simulink model "ThreeINVTRECT2025"  (R2024a)
settings: Solver=FixedStepAuto  StartTime=0.0  StopTime=0.3  FixedStep=2e-7  RelTol=1e-3
libraries: spsSeriesRLCBranchLib x27, spsCurrentMeasurementLib x5, spsUniversalBridgeLib x4, spsMeanLib x3, simulink x3, spsVoltageMeasurementLib x3, spsDCVoltageSourceLib x2, spsMutualInductanceLib x2, spsRMSLib x2, spsTHDLib x2, spspowerguiLib x1
settings Model: SimulationMode=accelerator  Creator=abc6820292  LastModifiedBy=50803
settings SolverCC: ZeroCrossControl=EnableAll  ZeroCrossAlgorithm=Adaptive
settings DebuggingCC: UnconnectedInputMsg=warning  UnconnectedOutputMsg=warning  UnconnectedLineMsg=warning
settings ModelReferenceCC: EnableRefExpFcnMdlSchedulingChecks=on
settings SFSimCC: SimTargetLang=C++
settings RTWCC: BuildConfiguration=Faster Runs  GPUComputeCapability=3.5  DLArmComputeVersion=19.05

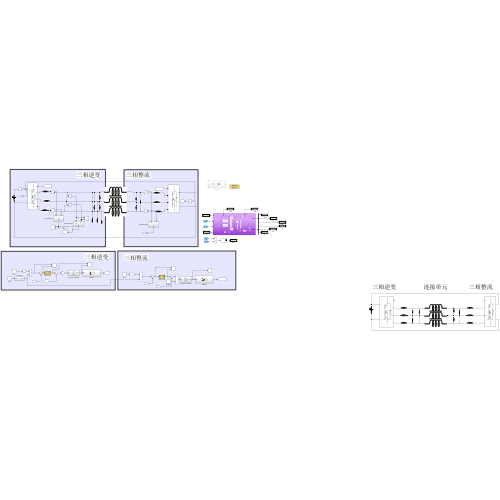
[thumbnail: Simulink's stored preview of the top-level diagram]
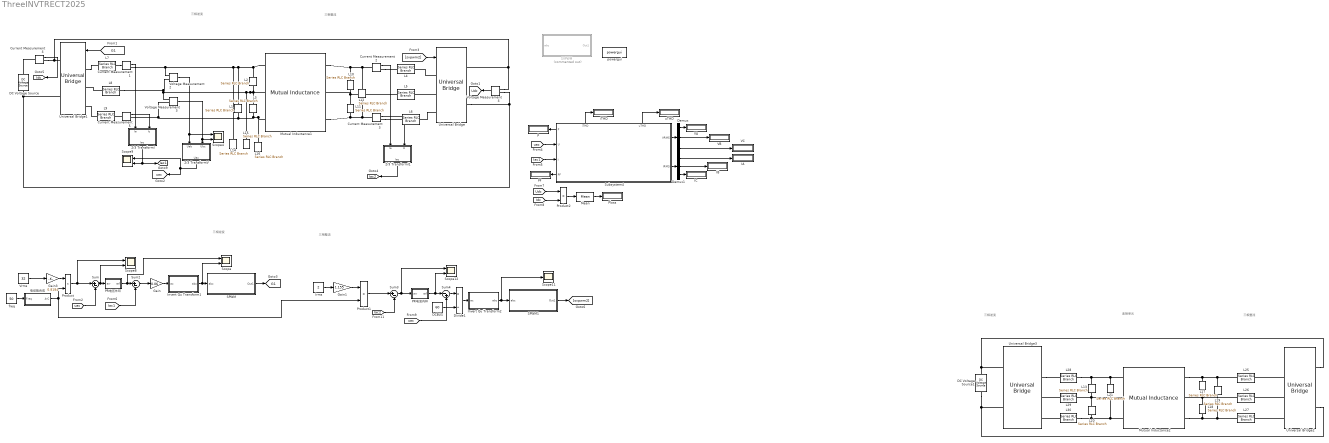
== system ThreeINVTRECT2025 ==
  note: 连接单元
  note: 三相逆变
  note: 三相逆变
  note: 三相整流
  note: 三相整流
  note: 三相逆变
  note: 三相整流
  2/3 TransformI : Subsystem
  2/3 TransformI1 : Subsystem
  2/3 TransformV : Subsystem
  Current Measurement{1..5} (5 alike) : spsCurrentMeasurementLib/Current Measurement  PhasorSimulation=off  OutputType=Complex  PSBequivalent=0
  DC Voltage Source : spsDCVoltageSourceLib/DC Voltage Source  Amplitude=60  Measurements=None
  DC Voltage Source1 : spsDCVoltageSourceLib/DC Voltage Source  Amplitude=60  Measurements=None
  DCBUS : Constant  Value=60
  Demux : Demux  Outputs=3
  Demux1 : Demux  Outputs=3
  Divide1 : Product  Inputs=*/
  Gain : Gain  Gain=0.06
  Gain1 : Gain  Gain=1.155
  Gain3 : Gain  Gain=0.8184
  IA : Display
      settings: Format=bank
  IB : Display
      settings: Format=bank
  IC : Display
      settings: Format=bank
  Invert Qu Transform1 : Subsystem
  Invert Qu Transform2 : Subsystem
  Irms : Constant  Value=2
  L{1..3,10..13,17..21} (12 alike) : spsSeriesRLCBranchLib/Series RLC Branch  LConnTagsString=__new0  RConnTagsString=__new0  BranchType=C  Resistance=16  Inductance=2e-3  SetiL0=off  InitialCurrent=0  Capacitance=2.2e-6  Setx0=off  InitialVoltage=0  Measurements=None
  L14 : spsSeriesRLCBranchLib/Series RLC Branch  LConnTagsString=__new0  RConnTagsString=__new0  BranchType=R  Resistance=16  Inductance=2e-3  SetiL0=off  InitialCurrent=0  Capacitance=2.2e-6  Setx0=off  InitialVoltage=0  Measurements=None
  L15 : spsSeriesRLCBranchLib/Series RLC Branch  LConnTagsString=__new0  RConnTagsString=__new0  BranchType=R  Resistance=16  Inductance=2e-3  SetiL0=off  InitialCurrent=0  Capacitance=2.2e-6  Setx0=off  InitialVoltage=0  Measurements=None
  L16 : spsSeriesRLCBranchLib/Series RLC Branch  LConnTagsString=__new0  RConnTagsString=__new0  BranchType=R  Resistance=16  Inductance=2e-3  SetiL0=off  InitialCurrent=0  Capacitance=2.2e-6  Setx0=off  InitialVoltage=0  Measurements=None
  L{4..9,25..30} (12 alike) : spsSeriesRLCBranchLib/Series RLC Branch  LConnTagsString=__new0  RConnTagsString=__new0  BranchType=L  Resistance=1  Inductance=7e-4  SetiL0=off  InitialCurrent=0  Capacitance=2e-3  Setx0=off  InitialVoltage=0  Measurements=None
  Mean : spsMeanLib/Mean  Freq=50  Vinit=0  Ts=0
  Mutual Inductance1 : spsMutualInductanceLib/Mutual Inductance  LConnTagsString=a|b|c  RConnTagsString=A|B|C  TypeOfMutual=Two or three windings with equal mutual terms  NumberOfWindings=3  SelfImpedance1=[0.01 1e-03]  SelfImpedance2=[0.01 1e-03]  ThreeWindings=on  SelfImpedance3=[0.01 1e-03]  MutualImpedance=[0.02 0.9e-03]  InductanceMatrix="[1.0 0.9  0.9 ;  0.9 1.0  0.9;  0.9 0.9 1.0 ] * 1e-3"  ResistanceMatrix="[1.0 0.9  0.9 ;  0.9 1.0  0.9;  0.9 0.9 1.0 ]"  Measurements=None
  Mutual Inductance2 : spsMutualInductanceLib/Mutual Inductance  LConnTagsString=a|b|c  RConnTagsString=A|B|C  TypeOfMutual=Two or three windings with equal mutual terms  NumberOfWindings=3  SelfImpedance1=[0.01 1e-03]  SelfImpedance2=[0.01 1e-03]  ThreeWindings=on  SelfImpedance3=[0.01 1e-03]  MutualImpedance=[0.02 0.9e-03]  InductanceMatrix="[1.0 0.9  0.9 ;  0.9 1.0  0.9;  0.9 0.9 1.0 ] * 1e-3"  ResistanceMatrix="[1.0 0.9  0.9 ;  0.9 1.0  0.9;  0.9 0.9 1.0 ]"  Measurements=None
  P : Display
      settings: Format=bank
  PF : Display
  PR电压外环 : Subsystem  TreatAsAtomicUnit=on  mask{Kp=1, Kr=50, Wc=5, Upper=80, Lower=-80}
  PR电流内环 : Subsystem  TreatAsAtomicUnit=on  mask{Kp=2, Kr=50, Wc=5, Upper=80, Lower=-80}
  Ploss : Display
  Product : Product
  Product1 : Product
  Product2 : Product
  SPWM : Subsystem
  SPWM1 : Subsystem
  SVPWM : Subsystem  Commented=on
  Scope{,4,8..9,12} (5 alike) : Scope  NumInputPorts=2
  Scope11 : Scope
  Subsystem4 : Subsystem
      settings: PortSchema="{\"entries\":[{\"content\":{\"sides\":[{\"content\":{\"connectorIds\":[\"Out5\",\"In1\",\"In2\",\"Out6\"]},\"type\":\"ConnectorPlacement.EquallySpacedRectSide\",\"uuid\":\"8f3b7bf1-7c44-4492-a357-aa6e3e6d66a4\"},{\"content\":{\"connectorIds\":[\"Out1\",\"Out2\"],\"side\":\"RIGHT\"},\"type\":\"ConnectorPlacement.EquallySpacedRectSide\",\"uuid\":\"7ae784cf-6bcf-4684-9c07-1770fc60c8a0\"},{\"content\":{\"connectorIds\":[\"Out3\",\"Out4\"],\"side\":\"TOP\"},\"type\":\"ConnectorPlacement.EquallySpacedRectSide\",\"uuid\":\"0e016931-6232-4ad6-afe9-572a0571336f\"},{\"content\":{\"side\":\"BOTTOM\"},\"type\":\"ConnectorPlacement.EquallySpacedRectSide\",\"uuid\":\"ef67c6ee-ba81-4705-af34-81581e7e9907\"}]},\"type\":\"ConnectorPlacement.EquallySpacedConnector\",\"uuid\":\"922af512-c0ff-443f-816c-194775a78dc8\"}],\"packageUris\":[\"http://schema.mathworks.com/mf0/Connector/R2020b\"],\"version\":\"1.0\"}"
  Sum : Sum  Inputs=|+-
  Sum2 : Sum  Inputs=|+-
  Sum3 : Sum  Inputs=|+-
  Sum4 : Sum  Inputs=|-+
  Universal Bridge{,1..3} (4 alike) : spsUniversalBridgeLib/Universal Bridge  Arms=3  SnubberResistance=1e5  SnubberCapacitance=inf  Device=MOSFET / Diodes  Ron=1e-3  Lon=0  ForwardVoltages="[  0  0  ]"  ForwardVoltage=0  GTOparameters=[ 10e-6 , 20e-6 ]  IGBTparameters=[ 1e-6 , 2e-6 ]  Measurements=None  Measurements_2=None  converterType=Rectifier
  VA : Display
      settings: Format=bank
  VB : Display
      settings: Format=bank
  VC : Display
      settings: Format=bank
  Voltage Measurement2 : spsVoltageMeasurementLib/Voltage Measurement  PhasorSimulation=off  OutputType=Complex  PSBequivalent=0
  Voltage Measurement3 : spsVoltageMeasurementLib/Voltage Measurement  PhasorSimulation=off  OutputType=Complex  PSBequivalent=0
  Voltage Measurement4 : spsVoltageMeasurementLib/Voltage Measurement  PhasorSimulation=off  OutputType=Complex  PSBequivalent=0
  Vrms : Constant  Value=32
  freq : Constant  Value=50
  iTHD : Display
  powergui : spspowerguiLib/powergui  SimulationMode=Discrete  SampleTime=2e-7  frequency=60  Iterations=50  frequencyindice=0  Pbase=100e6  ErrMax=1e-4  UnitsV=kV  UnitsW=MW  buscounter=0  FunctionMessages=off  echomessages=off  EnableUseOfTLC=off  CurrentSourceSwitches=off  DisableSnubberDevices=off  DisableRonSwitches=off  DisableVfSwitches=off  DisplayEquations=off  AutomaticDiscreteSolvers=off  SolverType=Tustin/Backward Euler (TBE)  Interpol=off  ExternalGateDelay=off  methode=off  Ts=0  x0status=blocks  SPID=off  SwTol=0  HookPort=off  NonlinearTolerance=1e-4  nMaxIteration=100  ContinueOnMaxIteration=off  RestoreLinks=warning  ResistiveCurrentMeasurement=off  Frange=[0:2:500]  Ylog=off  Xlog=on  ShowGrid=off  save=off  variable=ZData  structure=QQQQQ  ZoomFFT=off  StartTime=0.5  cycles=15  DisplayStyle=1  fundamental=50  FreqAxis=off  MaxFrequency=1000  frequencyindicesteady=1  RmsSteady=1  display=off
  uTHD : Display
  电动势合成 : Subsystem
      settings: PortSchema="{\"entries\":[{\"content\":{\"sides\":[{\"content\":{\"connectorIds\":[]},\"type\":\"ConnectorPlacement.EquallySpacedRectSide\",\"uuid\":\"ac756fcf-f6d7-466d-bb3d-287dec8ae983\"},{\"content\":{\"connectorIds\":[],\"side\":\"RIGHT\"},\"type\":\"ConnectorPlacement.EquallySpacedRectSide\",\"uuid\":\"3e1a0e91-a0b8-40c4-8839-5ebd84050a30\"},{\"content\":{\"connectorIds\":[\"In1\"],\"side\":\"TOP\"},\"type\":\"ConnectorPlacement.EquallySpacedRectSide\",\"uuid\":\"4c3986ff-483b-4975-8d50-1a8a46f35065\"},{\"content\":{\"connectorIds\":[\"Out1\"],\"side\":\"BOTTOM\"},\"type\":\"ConnectorPlacement.EquallySpacedRectSide\",\"uuid\":\"d0166e46-df65-4061-a961-140d500477a7\"}]},\"type\":\"ConnectorPlacement.EquallySpacedConnector\",\"uuid\":\"9d4b00aa-dfb1-427d-8698-7ec64c5ca012\"}],\"packageUris\":[\"http://schema.mathworks.com/mf0/Connector/R2020b\"],\"version\":\"1.0\"}"
  tag scope: G1=global, Iac1=global, Iac2=global, Idc=global, Udc=global, uac=global
  wires:
  [Iac1] -> Subsystem4/2(I)
  PR电流内环/1(ref) -> Sum4/1, Scope12/2
  [Iac2] -> Sum3/2
  Demux/3 -> VC/1
  [Iac1] -> Sum2/2
  Current Measurement5/1 -> 2/3 TransformI/2(Ic)
  Subsystem4/2(IRMS) -> Demux1/1
  2/3 TransformI/1(Iac) -> Scope9/2, [Iac1]
  [uac] -> Subsystem4/1(U)
  Subsystem4/1(VRMS) -> Demux/1
  Irms/1 -> Gain1/1
  Demux/2 -> VB/1
  2/3 TransformV/1(Uac) -> [uac], Scope9/1
  Demux/1 -> VA/1
  Subsystem4/5(P) -> P/1
  Demux1/3 -> IC/1
  SPWM1/1(Out1) -> [svpwm2]
  SPWM/1(Out1) -> [G1]
  Gain1/1 -> Product1/1
  Demux1/2 -> IB/1
  Current Measurement1/1 -> 2/3 TransformI/1(Ia)
  [G1] -> Universal Bridge1/1
  Voltage Measurement3/1 -> Scope4/2, 2/3 TransformV/2(Ubc)
  Subsystem4/6(PF) -> PF/1
  Sum3/1 -> PR电流内环/1(err), Scope12/1
  Invert Qu Transform2/1(abc) -> SPWM1/1(abc), Scope11/1
  Vrms/1 -> Gain3/1
  freq/1 -> 电动势合成/1(Freq)
  Demux1/1 -> IA/1
  Product1/1 -> Sum3/1
  电动势合成/1(A-C) -> Product/2, Product1/2
  [svpwm2] -> Universal Bridge/1
  Subsystem4/3(iTHD) -> iTHD/1
  Voltage Measurement2/1 -> Scope4/1, 2/3 TransformV/1(Uab)
  [uac] -> Sum/2
  Subsystem4/4(uTHD) -> uTHD/1
  Product/1 -> Scope8/1, Sum/1
  Voltage Measurement4/1 -> [Udc]
  Invert Qu Transform1/1(abc) -> Scope/2, SPWM/1(abc)
  Current Measurement2/1 -> 2/3 TransformI1/1(Ia)
  Current Measurement3/1 -> 2/3 TransformI1/2(Ic)
  2/3 TransformI1/1(Iac) -> [Iac2]
  Gain3/1 -> Product/1
  Current Measurement4/1 -> [Idc]
  [Idc] -> Product2/2
  [Udc] -> Product2/1
  Product2/1 -> Mean/1
  Mean/1 -> Ploss/1
  Divide1/1 -> Invert Qu Transform2/1(ac)
  Sum4/1 -> Divide1/1
  DCBUS/1 -> Divide1/2
  [uac] -> Sum4/2
  Sum/1 -> Scope8/2, PR电压外环/1(err)
  PR电压外环/1(ref) -> Scope/1, Sum2/1
  Gain/1 -> Invert Qu Transform1/1(ac)
  Sum2/1 -> Gain/1
  connections:
  L10/LConn1 -- Mutual Inductance1/RConn1 -- L12/LConn1 -- Current Measurement2/LConn1
  Current Measurement4/RConn1 -- Voltage Measurement4/LConn1 -- Universal Bridge/RConn1 -- Universal Bridge1/RConn1
  DC Voltage Source/LConn1 -- Universal Bridge1/RConn2 -- Universal Bridge/RConn2 -- Voltage Measurement4/LConn2
  Current Measurement5/RConn1 -- L16/LConn1 -- Mutual Inductance1/LConn3 -- L3/RConn1 -- L1/RConn1 -- Voltage Measurement3/LConn2
  Current Measurement3/RConn1 -- L6/LConn1
  L7/RConn1 -- Current Measurement1/LConn1
  Universal Bridge1/LConn1 -- L7/LConn1
  Universal Bridge/LConn3 -- L6/RConn1
  Universal Bridge/LConn2 -- L5/RConn1
  Current Measurement5/LConn1 -- L9/RConn1
  Current Measurement2/RConn1 -- L4/LConn1
  L9/LConn1 -- Universal Bridge1/LConn3
  Universal Bridge/LConn1 -- L4/RConn1
  L8/LConn1 -- Universal Bridge1/LConn2
  L5/LConn1 -- L11/LConn1 -- L10/RConn1 -- Mutual Inductance1/RConn2
  L14/LConn1 -- Current Measurement1/RConn1 -- Voltage Measurement2/LConn1 -- L1/LConn1 -- L2/LConn1 -- Mutual Inductance1/LConn1
  L3/LConn1 -- Mutual Inductance1/LConn2 -- L15/LConn1 -- L8/RConn1 -- Voltage Measurement2/LConn2 -- Voltage Measurement3/LConn1 -- L2/RConn1
  Current Measurement3/LConn1 -- Mutual Inductance1/RConn3 -- L11/RConn1 -- L12/RConn1
  DC Voltage Source/RConn1 -- Current Measurement4/LConn1
  Universal Bridge2/RConn1 -- DC Voltage Source1/RConn1 -- Universal Bridge3/RConn1
  L18/RConn1 -- L19/RConn1 -- L27/LConn1 -- Mutual Inductance2/RConn3
  Mutual Inductance2/RConn2 -- L18/LConn1 -- L26/LConn1 -- L17/RConn1
  Mutual Inductance2/RConn1 -- L25/LConn1 -- L19/LConn1 -- L17/LConn1
  Universal Bridge2/LConn1 -- L25/RConn1
  L30/RConn1 -- L20/RConn1 -- L21/RConn1 -- Mutual Inductance2/LConn3
  Universal Bridge2/LConn3 -- L27/RConn1
  L29/LConn1 -- Universal Bridge3/LConn2
  L30/LConn1 -- Universal Bridge3/LConn3
  Universal Bridge3/LConn1 -- L28/LConn1
  L28/RConn1 -- L13/LConn1 -- L21/LConn1 -- Mutual Inductance2/LConn1
  Universal Bridge2/LConn2 -- L26/RConn1
  DC Voltage Source1/LConn1 -- Universal Bridge2/RConn2 -- Universal Bridge3/RConn2
  Mutual Inductance2/LConn2 -- L13/RConn1 -- L20/LConn1 -- L29/RConn1

== system ThreeINVTRECT2025/2//3 TransformI ==
  Ia : Inport
  Ic : Inport  Port=2
  Mux : Mux  Inputs=2
  Iac : Outport
  wires:
  Ia/1 -> Mux/1
  Ic/1 -> Mux/2
  Mux/1 -> Iac/1

== system ThreeINVTRECT2025/2//3 TransformI1 ==
  Ia : Inport
  Ic : Inport  Port=2
  Mux : Mux  Inputs=2
  Iac : Outport
  wires:
  Mux/1 -> Iac/1
  Ic/1 -> Mux/2
  Ia/1 -> Mux/1

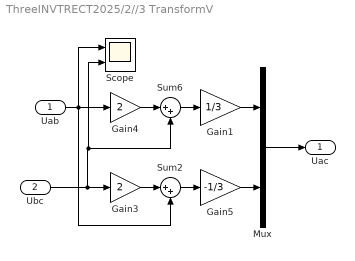
== system ThreeINVTRECT2025/2//3 TransformV ==
  Uab : Inport
  Ubc : Inport  Port=2
  Gain1 : Gain  Gain=1/3
  Gain3 : Gain  Gain=2
  Gain4 : Gain  Gain=2
  Gain5 : Gain  Gain=-1/3
  Mux : Mux  Inputs=2
  Scope : Scope  NumInputPorts=2
  Sum2 : Sum  Inputs=|++
  Sum6 : Sum  Inputs=|++
  Uac : Outport
  wires:
  Sum6/1 -> Gain1/1
  Uab/1 -> Scope/1, Sum2/2, Gain4/1
  Gain4/1 -> Sum6/1
  Ubc/1 -> Scope/2, Sum6/2, Gain3/1
  Gain3/1 -> Sum2/1
  Sum2/1 -> Gain5/1
  Gain5/1 -> Mux/2
  Gain1/1 -> Mux/1
  Mux/1 -> Uac/1

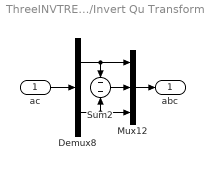
== system ThreeINVTRECT2025/Invert Qu Transform1 ==
  ac : Inport
  Demux8 : Demux  Outputs=2
  Mux12 : Mux  Inputs=3
  Sum2 : Sum  Inputs=-|-
  abc : Outport
  wires:
  Mux12/1 -> abc/1
  Demux8/2 -> Sum2/2, Mux12/3
  Sum2/1 -> Mux12/2
  ac/1 -> Demux8/1
  Demux8/1 -> Sum2/1, Mux12/1

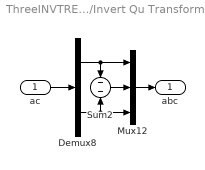
== system ThreeINVTRECT2025/Invert Qu Transform2 ==
  ac : Inport
  Demux8 : Demux  Outputs=2
  Mux12 : Mux  Inputs=3
  Sum2 : Sum  Inputs=-|-
  abc : Outport
  wires:
  Demux8/1 -> Mux12/1, Sum2/1
  ac/1 -> Demux8/1
  Sum2/1 -> Mux12/2
  Demux8/2 -> Mux12/3, Sum2/2
  Mux12/1 -> abc/1

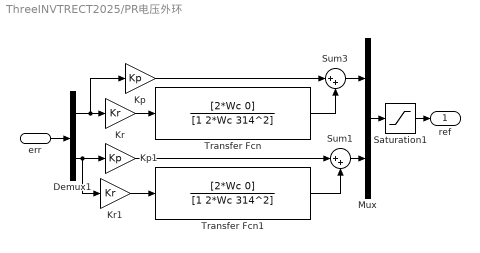
== system ThreeINVTRECT2025/PR电压外环 ==
  err : Inport
  Demux1 : Demux  Outputs=2
  Kp : Gain  Gain=Kp
  Kp1 : Gain  Gain=Kp
  Kr : Gain  Gain=Kr
  Kr1 : Gain  Gain=Kr
  Mux : Mux  Inputs=2
  Saturation1 : Saturate  UpperLimit=Upper  LowerLimit=Lower
  Sum1 : Sum  Inputs=|++
  Sum3 : Sum  Inputs=|++
  Transfer Fcn : TransferFcn  Numerator=[2*Wc 0]  Denominator=[1 2*Wc 314^2]
  Transfer Fcn1 : TransferFcn  Numerator=[2*Wc 0]  Denominator=[1 2*Wc 314^2]
  ref : Outport
  wires:
  Kp/1 -> Sum3/1
  Kr/1 -> Transfer Fcn/1
  Transfer Fcn/1 -> Sum3/2
  Demux1/1 -> Kp/1, Kr/1
  err/1 -> Demux1/1
  Demux1/2 -> Kr1/1, Kp1/1
  Kp1/1 -> Sum1/1
  Kr1/1 -> Transfer Fcn1/1
  Transfer Fcn1/1 -> Sum1/2
  Sum1/1 -> Mux/2
  Sum3/1 -> Mux/1
  Mux/1 -> Saturation1/1
  Saturation1/1 -> ref/1

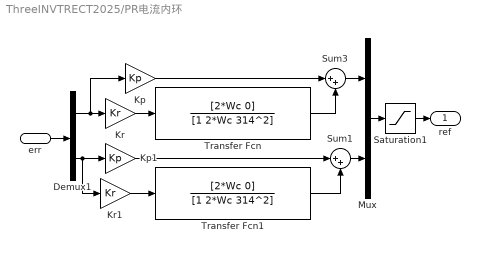
== system ThreeINVTRECT2025/PR电流内环 ==
  err : Inport
  Demux1 : Demux  Outputs=2
  Kp : Gain  Gain=Kp
  Kp1 : Gain  Gain=Kp
  Kr : Gain  Gain=Kr
  Kr1 : Gain  Gain=Kr
  Mux : Mux  Inputs=2
  Saturation1 : Saturate  UpperLimit=Upper  LowerLimit=Lower
  Sum1 : Sum  Inputs=|++
  Sum3 : Sum  Inputs=|++
  Transfer Fcn : TransferFcn  Numerator=[2*Wc 0]  Denominator=[1 2*Wc 314^2]
  Transfer Fcn1 : TransferFcn  Numerator=[2*Wc 0]  Denominator=[1 2*Wc 314^2]
  ref : Outport
  wires:
  Saturation1/1 -> ref/1
  Mux/1 -> Saturation1/1
  Sum3/1 -> Mux/1
  Sum1/1 -> Mux/2
  Transfer Fcn1/1 -> Sum1/2
  Kr1/1 -> Transfer Fcn1/1
  Kp1/1 -> Sum1/1
  Demux1/2 -> Kp1/1, Kr1/1
  err/1 -> Demux1/1
  Demux1/1 -> Kr/1, Kp/1
  Transfer Fcn/1 -> Sum3/2
  Kr/1 -> Transfer Fcn/1
  Kp/1 -> Sum3/1

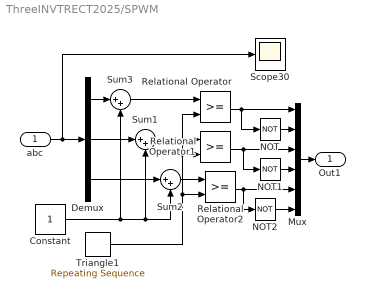
== system ThreeINVTRECT2025/SPWM ==
  abc : Inport
  Constant : Constant
  Demux : Demux  Outputs=3
  Mux : Mux  Inputs=6
  NOT : Logic  Operator=NOT  IconShape=distinctive  AllPortsSameDT=off  OutDataTypeStr=boolean
  NOT1 : Logic  Operator=NOT  IconShape=distinctive  AllPortsSameDT=off  OutDataTypeStr=boolean
  NOT2 : Logic  Operator=NOT  IconShape=distinctive  AllPortsSameDT=off  OutDataTypeStr=boolean
  Relational Operator : RelationalOperator  OutDataTypeStr=boolean  RndMeth=Simplest  InputSameDT=off
  Relational Operator1 : RelationalOperator  OutDataTypeStr=boolean  RndMeth=Simplest  InputSameDT=off
  Relational Operator2 : RelationalOperator  OutDataTypeStr=boolean  RndMeth=Simplest  InputSameDT=off
  Scope30 : Scope
  Sum1 : Sum  Inputs=|++
  Sum2 : Sum  Inputs=|++
  Sum3 : Sum  Inputs=|++
  Triangle1 : simulink/Sources/Repeating Sequence  rep_seq_t=[0 1/20000/2 1/20000]  rep_seq_y=[0 2 0]
  Out1 : Outport
  wires:
  Mux/1 -> Out1/1
  NOT2/1 -> Mux/6
  NOT1/1 -> Mux/4
  Relational Operator2/1 -> Mux/5, NOT2/1
  Relational Operator1/1 -> Mux/3, NOT1/1
  Relational Operator/1 -> Mux/1, NOT/1
  NOT/1 -> Mux/2
  Triangle1/1 -> Relational Operator/2, Relational Operator1/2, Relational Operator2/2
  abc/1 -> Scope30/1, Demux/1
  Demux/1 -> Sum3/1
  Sum3/1 -> Relational Operator/1
  Demux/2 -> Sum1/1
  Sum1/1 -> Relational Operator1/1
  Demux/3 -> Sum2/1
  Sum2/1 -> Relational Operator2/1
  Constant/1 -> Sum2/2, Sum1/2, Sum3/2

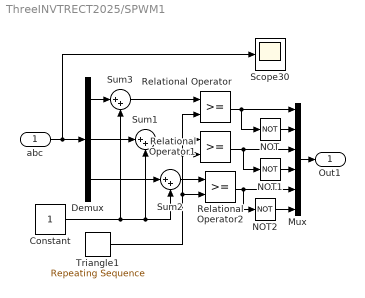
== system ThreeINVTRECT2025/SPWM1 ==
  abc : Inport
  Constant : Constant
  Demux : Demux  Outputs=3
  Mux : Mux  Inputs=6
  NOT : Logic  Operator=NOT  IconShape=distinctive  AllPortsSameDT=off  OutDataTypeStr=boolean
  NOT1 : Logic  Operator=NOT  IconShape=distinctive  AllPortsSameDT=off  OutDataTypeStr=boolean
  NOT2 : Logic  Operator=NOT  IconShape=distinctive  AllPortsSameDT=off  OutDataTypeStr=boolean
  Relational Operator : RelationalOperator  OutDataTypeStr=boolean  RndMeth=Simplest  InputSameDT=off
  Relational Operator1 : RelationalOperator  OutDataTypeStr=boolean  RndMeth=Simplest  InputSameDT=off
  Relational Operator2 : RelationalOperator  OutDataTypeStr=boolean  RndMeth=Simplest  InputSameDT=off
  Scope30 : Scope
  Sum1 : Sum  Inputs=|++
  Sum2 : Sum  Inputs=|++
  Sum3 : Sum  Inputs=|++
  Triangle1 : simulink/Sources/Repeating Sequence  rep_seq_t=[0 1/20000/2 1/20000]  rep_seq_y=[0 2 0]
  Out1 : Outport
  wires:
  Constant/1 -> Sum3/2, Sum1/2, Sum2/2
  Sum2/1 -> Relational Operator2/1
  Demux/3 -> Sum2/1
  Sum1/1 -> Relational Operator1/1
  Demux/2 -> Sum1/1
  Sum3/1 -> Relational Operator/1
  Demux/1 -> Sum3/1
  abc/1 -> Demux/1, Scope30/1
  Triangle1/1 -> Relational Operator2/2, Relational Operator1/2, Relational Operator/2
  NOT/1 -> Mux/2
  Relational Operator/1 -> NOT/1, Mux/1
  Relational Operator1/1 -> NOT1/1, Mux/3
  Relational Operator2/1 -> NOT2/1, Mux/5
  NOT1/1 -> Mux/4
  NOT2/1 -> Mux/6
  Mux/1 -> Out1/1

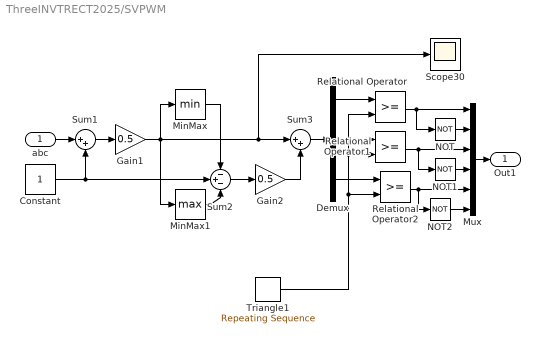
== system ThreeINVTRECT2025/SVPWM ==
  abc : Inport
  Constant : Constant
  Demux : Demux  Outputs=3
  Gain1 : Gain  Gain=0.5
  Gain2 : Gain  Gain=0.5
  MinMax : MinMax
  MinMax1 : MinMax  Function=max
  Mux : Mux  Inputs=6
  NOT : Logic  Operator=NOT  IconShape=distinctive  AllPortsSameDT=off  OutDataTypeStr=boolean
  NOT1 : Logic  Operator=NOT  IconShape=distinctive  AllPortsSameDT=off  OutDataTypeStr=boolean
  NOT2 : Logic  Operator=NOT  IconShape=distinctive  AllPortsSameDT=off  OutDataTypeStr=boolean
  Relational Operator : RelationalOperator  OutDataTypeStr=boolean  RndMeth=Simplest  InputSameDT=off
  Relational Operator1 : RelationalOperator  OutDataTypeStr=boolean  RndMeth=Simplest  InputSameDT=off
  Relational Operator2 : RelationalOperator  OutDataTypeStr=boolean  RndMeth=Simplest  InputSameDT=off
  Scope30 : Scope
  Sum1 : Sum  Inputs=|++
  Sum2 : Sum  Inputs=-+-
  Sum3 : Sum  Inputs=|++
  Triangle1 : simulink/Sources/Repeating Sequence  rep_seq_t=[0 1/20000/2 1/20000]  rep_seq_y=[0 1 0]
  Out1 : Outport
  wires:
  abc/1 -> Sum1/1
  Sum1/1 -> Gain1/1
  Constant/1 -> Sum1/2, Sum2/2
  MinMax/1 -> Sum2/1
  Gain1/1 -> Scope30/1, Sum3/1, MinMax1/1, MinMax/1
  MinMax1/1 -> Sum2/3
  Sum2/1 -> Gain2/1
  Gain2/1 -> Sum3/2
  Sum3/1 -> Demux/1
  Demux/2 -> Relational Operator1/1
  Demux/1 -> Relational Operator/1
  Demux/3 -> Relational Operator2/1
  Triangle1/1 -> Relational Operator/2, Relational Operator1/2, Relational Operator2/2
  NOT/1 -> Mux/2
  Relational Operator/1 -> NOT/1, Mux/1
  Relational Operator1/1 -> NOT1/1, Mux/3
  Relational Operator2/1 -> NOT2/1, Mux/5
  NOT1/1 -> Mux/4
  NOT2/1 -> Mux/6
  Mux/1 -> Out1/1

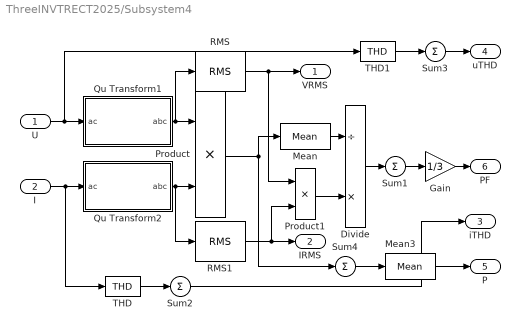
== system ThreeINVTRECT2025/Subsystem4 ==
  U : Inport
  I : Inport  Port=2
  Divide : Product  Inputs=/*
  Gain : Gain  Gain=1/3
  Mean : spsMeanLib/Mean  Freq=50  Vinit=0  Ts=0
  Mean3 : spsMeanLib/Mean  Freq=50  Vinit=0  Ts=0
  Product : Product
  Product1 : Product
  Qu Transform1 : Subsystem
  Qu Transform2 : Subsystem
  RMS : spsRMSLib/RMS  TrueRMS=on  Freq=50  RMSInit=0  Ts=0
  RMS1 : spsRMSLib/RMS  TrueRMS=on  Freq=50  RMSInit=0  Ts=0
  Sum{1..4} (4 alike) : Sum  Inputs=+
  THD : spsTHDLib/THD  Freq=50  Ts=0
  THD1 : spsTHDLib/THD  Freq=50  Ts=0
  VRMS : Outport
  IRMS : Outport  Port=2
  iTHD : Outport  Port=3
  uTHD : Outport  Port=4
  P : Outport  Port=5
  PF : Outport  Port=6
  wires:
  RMS/1 -> Product1/1, VRMS/1
  Gain/1 -> PF/1
  Mean3/1 -> P/1
  Qu Transform1/1(abc) -> Product/1, RMS/1
  U/1 -> THD1/1, Qu Transform1/1(ac)
  I/1 -> THD/1, Qu Transform2/1(ac)
  Qu Transform2/1(abc) -> Product/2, RMS1/1
  THD/1 -> Sum2/1
  THD1/1 -> Sum3/1
  Product/1 -> Sum4/1, Mean/1
  Sum4/1 -> Mean3/1
  RMS1/1 -> Product1/2, IRMS/1
  Product1/1 -> Divide/2
  Mean/1 -> Divide/1
  Divide/1 -> Sum1/1
  Sum1/1 -> Gain/1
  Sum3/1 -> uTHD/1
  Sum2/1 -> iTHD/1

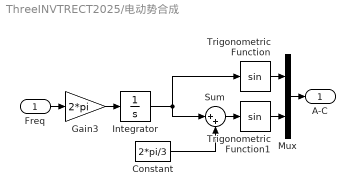
== system ThreeINVTRECT2025/电动势合成 ==
  Freq : Inport
  Constant : Constant  Value=2*pi/3
  Gain3 : Gain  Gain=2*pi
  Integrator : Integrator  WrapState=on  WrappedStateUpperValue=2*pi  WrappedStateLowerValue=0
  Mux : Mux  Inputs=2
  Sum : Sum  Inputs=|++
  Trigonometric Function : Trigonometry
  Trigonometric Function1 : Trigonometry
  A-C : Outport
  wires:
  Gain3/1 -> Integrator/1
  Mux/1 -> A-C/1
  Trigonometric Function/1 -> Mux/1
  Trigonometric Function1/1 -> Mux/2
  Sum/1 -> Trigonometric Function1/1
  Constant/1 -> Sum/2
  Integrator/1 -> Sum/1, Trigonometric Function/1
  Freq/1 -> Gain3/1

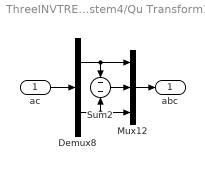
== system ThreeINVTRECT2025/Subsystem4/Qu Transform1 ==
  ac : Inport
  Demux8 : Demux  Outputs=2
  Mux12 : Mux  Inputs=3
  Sum2 : Sum  Inputs=-|-
  abc : Outport
  wires:
  Mux12/1 -> abc/1
  Demux8/2 -> Sum2/2, Mux12/3
  Sum2/1 -> Mux12/2
  ac/1 -> Demux8/1
  Demux8/1 -> Sum2/1, Mux12/1

== system ThreeINVTRECT2025/Subsystem4/Qu Transform2 ==
  ac : Inport
  Demux8 : Demux  Outputs=2
  Mux12 : Mux  Inputs=3
  Sum2 : Sum  Inputs=-|-
  abc : Outport
  wires:
  Demux8/1 -> Mux12/1, Sum2/1
  ac/1 -> Demux8/1
  Sum2/1 -> Mux12/2
  Demux8/2 -> Mux12/3, Sum2/2
  Mux12/1 -> abc/1
